simulink model "BPSK_QPSK_AWGN_BER"  (Simulink 10.1)
settings: Solver=FixedStepDiscrete  StartTime=0.0  StopTime=1e6*2e-005  RelTol=1e-3  EnableMultiTasking=on
PreLoadFcn:
  | bitRate = 500000;
  | bitsPerFrame = 200;
  | maxDopplerShift = 200;
  | delayVector = [0:3]*(4e-6);
  | gainVector = [0:3]*(-3);
  | LOSDopplerShift = 100;
  | KFactor = 10;
libraries: commdigbbndam3 x6, commchan3 x4, commsink2 x4, commcnvcod2 x3, commrandsrc2 x1
Description:
  | Multipath Fading Channel
  | 
  | To learn about this model, click <a href="matlab: showdemo multipathfading_demo;">here</a>.
CloseFcn:
  | clear bitRate
  | clear bitsPerFrame
  | clear maxDopplerShift
  | clear delayVector
  | clear gainVector
  | clear LOSDopplerShift
  | clear KFactor
settings Model: Creator=The MathWorks Inc.  LastModifiedBy=Administrator  ExtModeAutoUpdateStatusClock=off
settings DataIOCC: SignalLoggingSaveFormat=ModelDataLogs  SaveOutput=off  SignalLogging=off  SaveTime=off  SignalLoggingName=multipathSigsOut
settings OptimizationCC: BooleanDataType=off  OptimizeBlockIOStorage=off  BufferReuse=off  GlobalBufferReuse=off  ExpressionFolding=off  ExpressionDepthLimit=2147483647  LocalBlockOutputs=off  InitFltsAndDblsToZero=on  BufferReusableBoundary=off  OptimizeDataStoreBuffers=off  BusAssignmentInplaceUpdate=off
settings DebuggingCC: SaveWithParameterizedLinksMsg=none  CheckExecutionContextPreStartOutputMsg=on  CheckExecutionContextRuntimeOutputMsg=on  SignalResolutionControl=TryResolveAllWithWarning  InheritedTsInSrcMsg=none  MultiTaskDSMMsg=warning  MultiTaskCondExecSysMsg=none  SigSpecEnsureSampleTimeMsg=none  FcnCallInpInsideContextMsg=warning  BusObjectLabelMismatch=none  StateNameClashWarn=warning
settings HardwareCC: TargetUnknown=on
settings ModelReferenceCC: UpdateModelReferenceTargets=IfOutOfDate
settings GRTTargetCC: TargetFcnLib=ansi_tfl_tmw.mat

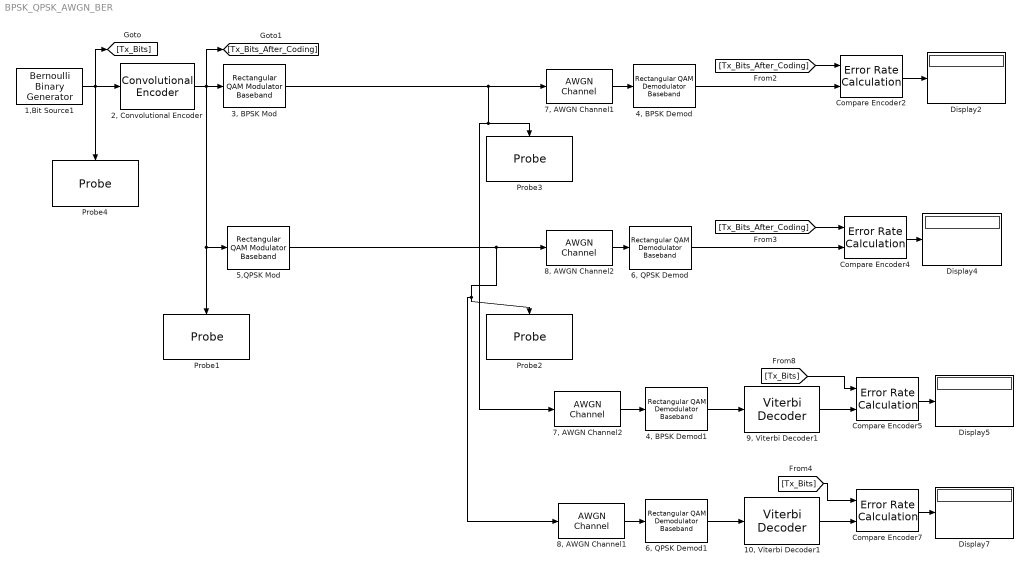
== system BPSK_QPSK_AWGN_BER ==
  1,Bit Source1 : commrandsrc2/Bernoulli Binary Generator  P=0.5  seed=61  Ts=2e-006  frameBased=on  sampPerFrame=8  orient=off  outDataType=double
      settings: SourceProductBaseCode=CM
  "10, Viterbi Decoder1" : commcnvcod2/Viterbi Decoder  trellis=poly2trellis(7, [171 133])  isPunctured=off  punctureVector=[1; 1; 0; 1; 0; 1]  erasures=off  dectype=Hard decision  nsdecb=4  runSigValErrCheck=off  tbdepth=34  opmode=Continuous  reset=off  delayedResetAction=off  smWordLength=16  outDataType=Inherit via internal rule
      settings: SourceProductBaseCode=CM
  "2, Convolutional Encoder" : commcnvcod2/Convolutional Encoder  trellis=poly2trellis(7, [171 133])  opMode=Continuous  DelayedResetAction=off  hasIniStPort=off  hasFinStPort=off  usePuncVector=off  punctureVector=[1; 1; 0; 1; 0; 1]  reset=Unused parameter value
      settings: SourceProductBaseCode=CM
  "3, BPSK Mod" : commdigbbndam3/Rectangular QAM Modulator Baseband  M=2  InType=Bit  Enc=Gray  Mapping=[0,1,2,3]  PowType=Average Power  MinDist=2  AvgPow=1  PeakPow=1  Ph=0  outDtype=double  outWordLen=16  outUDDataType=sfix(16)  outFracLenMode=Best precision  outFracLen=15  outDataTypeStr=double  outLastDataTypeStr=double
  "4, BPSK Demod" : commdigbbndam3/Rectangular QAM Demodulator Baseband  M=2  OutType=Bit  DecType=Hard decision  VarSource=Dialog  Variance=1  Dec=Gray  Mapping=[0:15]  PowType=Average Power  MinDist=2  AvgPow=1  PeakPow=1  Ph=0  outDtype1=Inherit via internal rule  outDtype2=Inherit via internal rule  derotateFactorWordLen=16  derotateFactorDataTypeStr=Inherit: Same word length as input  derotateFactorLastDataTypeStr=Inherit: Same word length as input  denormFactorWordLen=16  denormFactorDataTypeStr=Inherit: Same word length as input  denormFactorLastDataTypeStr=Inherit: Same word length as input  prodOutWordLen=32  prodOutOverflowMode=Wrap  prodOutRoundingMode=Floor  prodOutOvFlMode=off  prodOutOvFlModeLastStrValue=off  sumWordLen=32
  "4, BPSK Demod1" : commdigbbndam3/Rectangular QAM Demodulator Baseband  M=2  OutType=Bit  DecType=Hard decision  VarSource=Dialog  Variance=1  Dec=Gray  Mapping=[0:15]  PowType=Average Power  MinDist=2  AvgPow=1  PeakPow=1  Ph=0  outDtype1=Inherit via internal rule  outDtype2=Inherit via internal rule  derotateFactorWordLen=16  derotateFactorDataTypeStr=Inherit: Same word length as input  derotateFactorLastDataTypeStr=Inherit: Same word length as input  denormFactorWordLen=16  denormFactorDataTypeStr=Inherit: Same word length as input  denormFactorLastDataTypeStr=Inherit: Same word length as input  prodOutWordLen=32  prodOutOverflowMode=Wrap  prodOutRoundingMode=Floor  prodOutOvFlMode=off  prodOutOvFlModeLastStrValue=off  sumWordLen=32
  5,QPSK Mod : commdigbbndam3/Rectangular QAM Modulator Baseband  M=4  InType=Bit  Enc=Gray  Mapping=[0,1,2,3]  PowType=Average Power  MinDist=2  AvgPow=1  PeakPow=1  Ph=-pi/2  outDtype=double  outWordLen=16  outUDDataType=sfix(16)  outFracLenMode=Best precision  outFracLen=15  outDataTypeStr=double  outLastDataTypeStr=double
  "6, QPSK Demod" : commdigbbndam3/Rectangular QAM Demodulator Baseband  M=4  OutType=Bit  DecType=Hard decision  VarSource=Dialog  Variance=1  Dec=Gray  Mapping=[0:15]  PowType=Average Power  MinDist=2  AvgPow=1  PeakPow=1  Ph=-pi/2  outDtype1=Inherit via internal rule  outDtype2=Inherit via internal rule  derotateFactorWordLen=16  derotateFactorDataTypeStr=Inherit: Same word length as input  derotateFactorLastDataTypeStr=Inherit: Same word length as input  denormFactorWordLen=16  denormFactorDataTypeStr=Inherit: Same word length as input  denormFactorLastDataTypeStr=Inherit: Same word length as input  prodOutWordLen=32  prodOutOverflowMode=Wrap  prodOutRoundingMode=Floor  prodOutOvFlMode=off  prodOutOvFlModeLastStrValue=off  sumWordLen=32
  "6, QPSK Demod1" : commdigbbndam3/Rectangular QAM Demodulator Baseband  M=4  OutType=Bit  DecType=Hard decision  VarSource=Dialog  Variance=1  Dec=Gray  Mapping=[0:15]  PowType=Average Power  MinDist=2  AvgPow=1  PeakPow=1  Ph=-pi/2  outDtype1=Inherit via internal rule  outDtype2=Inherit via internal rule  derotateFactorWordLen=16  derotateFactorDataTypeStr=Inherit: Same word length as input  derotateFactorLastDataTypeStr=Inherit: Same word length as input  denormFactorWordLen=16  denormFactorDataTypeStr=Inherit: Same word length as input  denormFactorLastDataTypeStr=Inherit: Same word length as input  prodOutWordLen=32  prodOutOverflowMode=Wrap  prodOutRoundingMode=Floor  prodOutOvFlMode=off  prodOutOvFlModeLastStrValue=off  sumWordLen=32
  "7, AWGN Channel1" : commchan3/AWGN Channel  InputProcessing=Columns as channels (frame based)  seed=67  noiseMode="Signal to noise ratio  (Es/No)"  EbNodB=5  EsNodB=6.5  SNRdB=10  bitsPerSym=1  Ps=1  Tsym=1.0000e-006  variance=1
  "7, AWGN Channel2" : commchan3/AWGN Channel  InputProcessing=Columns as channels (frame based)  seed=67  noiseMode="Signal to noise ratio  (Es/No)"  EbNodB=5  EsNodB=6.5-3  SNRdB=10  bitsPerSym=1  Ps=1  Tsym=1.0000e-006  variance=1
  "8, AWGN Channel1" : commchan3/AWGN Channel  InputProcessing=Columns as channels (frame based)  seed=67  noiseMode="Signal to noise ratio  (Es/No)"  EbNodB=5  EsNodB=6  SNRdB=10  bitsPerSym=2  Ps=1  Tsym=1.0000e-006*2  variance=1
  "8, AWGN Channel2" : commchan3/AWGN Channel  InputProcessing=Columns as channels (frame based)  seed=67  noiseMode="Signal to noise ratio  (Es/No)"  EbNodB=5  EsNodB=6+3  SNRdB=10  bitsPerSym=2  Ps=1  Tsym=1.0000e-006*2  variance=1
  "9, Viterbi Decoder1" : commcnvcod2/Viterbi Decoder  trellis=poly2trellis(7, [171 133])  isPunctured=off  punctureVector=[1; 1; 0; 1; 0; 1]  erasures=off  dectype=Hard decision  nsdecb=4  runSigValErrCheck=off  tbdepth=34  opmode=Continuous  reset=off  delayedResetAction=off  smWordLength=16  outDataType=Inherit via internal rule
      settings: SourceProductBaseCode=CM
  Compare Encoder2 : commsink2/Error Rate Calculation  N=0  st_delay=0  cp_mode=Entire frame  subframe=[]  PMode=Port  WsName=ErrorVec  RsMode2=off  stop=off  numErr=100  maxBits=1e6
  Compare Encoder4 : commsink2/Error Rate Calculation  N=0  st_delay=0  cp_mode=Entire frame  subframe=[]  PMode=Port  WsName=ErrorVec  RsMode2=off  stop=off  numErr=100  maxBits=1e6
  Compare Encoder5 : commsink2/Error Rate Calculation  N=34  st_delay=0  cp_mode=Entire frame  subframe=[]  PMode=Port  WsName=ErrorVec  RsMode2=off  stop=off  numErr=100  maxBits=1e6
  Compare Encoder7 : commsink2/Error Rate Calculation  N=34  st_delay=0  cp_mode=Entire frame  subframe=[]  PMode=Port  WsName=ErrorVec  RsMode2=off  stop=off  numErr=100  maxBits=1e6
  Display{2,4..5,7} (4 alike) : Display
  Probe{1..4} (4 alike) : Probe  ProbeComplexSignal=off  ProbeSampleTimeDataType=Same as input
  wires:
  "2, Convolutional Encoder"/1 -> [Tx_Bits_After_Coding], Probe1/1, 5,QPSK Mod/1, "3, BPSK Mod"/1
  "3, BPSK Mod"/1 -> Probe3/1, "7, AWGN Channel2"/1, "7, AWGN Channel1"/1
  "4, BPSK Demod"/1 -> Compare Encoder2/2
  "7, AWGN Channel1"/1 -> "4, BPSK Demod"/1
  Compare Encoder2/1 -> Display2/1
  5,QPSK Mod/1 -> "8, AWGN Channel2"/1, Probe2/1, "8, AWGN Channel1"/1
  "6, QPSK Demod"/1 -> Compare Encoder4/2
  "8, AWGN Channel2"/1 -> "6, QPSK Demod"/1
  Compare Encoder4/1 -> Display4/1
  1,Bit Source1/1 -> "2, Convolutional Encoder"/1, [Tx_Bits], Probe4/1
  [Tx_Bits_After_Coding] -> Compare Encoder2/1
  [Tx_Bits_After_Coding] -> Compare Encoder4/1
  "4, BPSK Demod1"/1 -> "9, Viterbi Decoder1"/1
  "9, Viterbi Decoder1"/1 -> Compare Encoder5/2
  Compare Encoder5/1 -> Display5/1
  "7, AWGN Channel2"/1 -> "4, BPSK Demod1"/1
  "6, QPSK Demod1"/1 -> "10, Viterbi Decoder1"/1
  "10, Viterbi Decoder1"/1 -> Compare Encoder7/2
  Compare Encoder7/1 -> Display7/1
  "8, AWGN Channel1"/1 -> "6, QPSK Demod1"/1
  [Tx_Bits] -> Compare Encoder5/1
  [Tx_Bits] -> Compare Encoder7/1
